simulink library "wt_blockset_v3"  (Simulink 6.0)
settings: Solver=ode45  SolverMode=SingleTasking  StartTime=0.0  StopTime=10.0  RelTol=1e-3
undefined symbols (not defined in the file): f1, get, j, Kmode, Type, u0
libraries: simulink_extras x12, simulink3 x5, simulink x4, dspinverses x1, dspmtrx3 x1, dspsnks4 x1
(part 5 of 7)

== system wt_blockset_v3/Mechanical Components/Wind Model ZA-1/Kaimal_Filter_2 ==
  in_1 : Inport  Port=1  LatchInput=off
  Gain : Gain  Gain=trans/sqrt(2)  SaturateOnIntegerOverflow=on
  Transfer Function : TransferFcn  Numerator=[0.0182*c^2 1.3653*c 0.9846]  Denominator=[1.3463*c^2 3.7593*c 1]
  Unit Delay : UnitDelay  SampleTime=T_sample
  out_1 : Outport
  wires:
  Unit Delay/1 -> Transfer Function/1
  Gain/1 -> out_1/1
  in_1/1 -> Unit Delay/1
  Transfer Function/1 -> Gain/1

== system wt_blockset_v3/Mechanical Components/Wind Model ZA-1/Kaimal_Filter_3 ==
  in_1 : Inport  Port=1  LatchInput=off
  Gain : Gain  Gain=trans/sqrt(2)  SaturateOnIntegerOverflow=on
  Transfer Fcn : TransferFcn  Numerator=[0.0182*c^2 1.3653*c 0.9846]  Denominator=[1.3463*c^2 3.7593*c 1]
  Unit Delay : UnitDelay  SampleTime=T_sample
  out_1 : Outport
  wires:
  Unit Delay/1 -> Transfer Fcn/1
  Gain/1 -> out_1/1
  in_1/1 -> Unit Delay/1
  Transfer Fcn/1 -> Gain/1

== system wt_blockset_v3/Mechanical Components/Wind Model ZA-2/3rd_Harmonic_Filter1 ==
  avg_wind : Inport  Port=1  LatchInput=off
  in_1 : Inport  Port=2  LatchInput=off
  3rd harmonic Filter : Subsystem
  Unit Delay : UnitDelay  SampleTime=T_sample
  out_1 : Outport
  wires:
  Unit Delay/1 -> 3rd harmonic Filter/2(In)
  in_1/1 -> Unit Delay/1
  avg_wind/1 -> 3rd harmonic Filter/1(avg_wind)
  3rd harmonic Filter/1(Out) -> out_1/1

== system wt_blockset_v3/Mechanical Components/Wind Model ZA-2/3rd_Harmonic_Filter2 ==
  avg_wind : Inport  Port=1  LatchInput=off
  in_1 : Inport  Port=2  LatchInput=off
  3rd harmonic Filter : Subsystem
  Unit Delay : UnitDelay  SampleTime=T_sample
  out_1 : Outport
  wires:
  3rd harmonic Filter/1(Out) -> out_1/1
  avg_wind/1 -> 3rd harmonic Filter/1(avg_wind)
  in_1/1 -> Unit Delay/1
  Unit Delay/1 -> 3rd harmonic Filter/2(In)

== system wt_blockset_v3/Mechanical Components/Wind Model ZA-2/Band Limited White Noise ==
  Gain : Gain  Gain=sqrt(noise/T_sample)  SaturateOnIntegerOverflow=on
  S-Function : S-Function  FunctionName=rngen  Parameters=seed
  Zero-Order Hold : ZeroOrderHold  SampleTime=T_sample
  wn : Outport
  wires:
  S-Function/1 -> Zero-Order Hold/1
  Zero-Order Hold/1 -> Gain/1
  Gain/1 -> wn/1

== system wt_blockset_v3/Mechanical Components/Wind Model ZA-2/Band Limited White Noise1 ==
  Gain : Gain  Gain=sqrt(noise/T_sample)  SaturateOnIntegerOverflow=on
  S-Function : S-Function  FunctionName=rngen  Parameters=seed
  Zero-Order Hold : ZeroOrderHold  SampleTime=T_sample
  wn : Outport
  wires:
  Gain/1 -> wn/1
  Zero-Order Hold/1 -> Gain/1
  S-Function/1 -> Zero-Order Hold/1

== system wt_blockset_v3/Mechanical Components/Wind Model ZA-2/Band Limited White Noise2 ==
  Gain : Gain  Gain=sqrt(noise/T_sample)  SaturateOnIntegerOverflow=on
  S-Function : S-Function  FunctionName=rngen  Parameters=seed
  Zero-Order Hold : ZeroOrderHold  SampleTime=T_sample
  wn : Outport
  wires:
  S-Function/1 -> Zero-Order Hold/1
  Zero-Order Hold/1 -> Gain/1
  Gain/1 -> wn/1

== system wt_blockset_v3/Mechanical Components/Wind Model ZA-2/Kaimal_Filter_1 ==
  in_1 : Inport  Port=1  LatchInput=off
  avg_wind : Inport  Port=2  LatchInput=off
  Fcn : Fcn  Expr=turb_int*sqrt(L*u(1))/100/sqrt(2)
  Kaimal Filter : Subsystem
  Product : Product  SaturateOnIntegerOverflow=on
  Unit Delay : UnitDelay  SampleTime=T_sample
  out_1 : Outport
  wires:
  Unit Delay/1 -> Kaimal Filter/2(In)
  in_1/1 -> Unit Delay/1
  avg_wind/1 -> Kaimal Filter/1(avg_wind), Fcn/1
  Fcn/1 -> Product/1
  Kaimal Filter/1(Out) -> Product/2
  Product/1 -> out_1/1

== system wt_blockset_v3/Mechanical Components/Wind Model ZA-2/Kaimal_Filter_2 ==
  avg_wind : Inport  Port=1  LatchInput=off
  in_1 : Inport  Port=2  LatchInput=off
  Fcn : Fcn  Expr=turb_int*sqrt(L*u(1))/100/sqrt(2)
  Kaimal Filter : Subsystem
  Product : Product  SaturateOnIntegerOverflow=on
  Unit Delay : UnitDelay  SampleTime=T_sample
  out_1 : Outport
  wires:
  Product/1 -> out_1/1
  Kaimal Filter/1(Out) -> Product/2
  Fcn/1 -> Product/1
  avg_wind/1 -> Fcn/1, Kaimal Filter/1(avg_wind)
  in_1/1 -> Unit Delay/1
  Unit Delay/1 -> Kaimal Filter/2(In)

== system wt_blockset_v3/Mechanical Components/Wind Model ZA-2/Kaimal_Filter_3 ==
  avg_wind : Inport  Port=1  LatchInput=off
  in_1 : Inport  Port=2  LatchInput=off
  Fcn : Fcn  Expr=turb_int*sqrt(L*u(1))/100/sqrt(2)
  Kaimal Filter : Subsystem
  Product : Product  SaturateOnIntegerOverflow=on
  Unit Delay : UnitDelay  SampleTime=T_sample
  out_1 : Outport
  wires:
  Unit Delay/1 -> Kaimal Filter/2(In)
  in_1/1 -> Unit Delay/1
  avg_wind/1 -> Kaimal Filter/1(avg_wind), Fcn/1
  Fcn/1 -> Product/1
  Kaimal Filter/1(Out) -> Product/2
  Product/1 -> out_1/1

== system wt_blockset_v3/Mechanical Components/Wind Model ZA-2/ZERO_Harmonic_Filter ==
  in_1 : Inport  Port=1  LatchInput=off
  avg_wind : Inport  Port=2  LatchInput=off
  Unit Delay : UnitDelay  SampleTime=T_sample
  ZERO harmonic Filter : Subsystem
  out_1 : Outport
  wires:
  ZERO harmonic Filter/1(Out) -> out_1/1
  avg_wind/1 -> ZERO harmonic Filter/1(avg_wind)
  in_1/1 -> Unit Delay/1
  Unit Delay/1 -> ZERO harmonic Filter/2(In)

== system wt_blockset_v3/Power Converters/3-phase Diode Bridge Rectifier/Diode  State Calculator ==
  note: K = [d1 - d4
      |        d3 - d6
      |         d5 - d2]
  RST : Inport  Port=1  LatchInput=off
  Branch A+ : Subsystem
  Branch A- : Subsystem
  Branch B+ : Subsystem
  Branch B- : Subsystem
  Branch C+ : Subsystem
  Branch C- : Subsystem
  Mux : Mux  Inputs=3
  Sum : Sum  Inputs=+-  SaturateOnIntegerOverflow=on  InputSameDT=on
  Sum1 : Sum  Inputs=+-  SaturateOnIntegerOverflow=on  InputSameDT=on
  Sum2 : Sum  Inputs=+-  SaturateOnIntegerOverflow=on  InputSameDT=on
  K : Outport  InitialOutput=0
  wires:
  RST/1 -> Branch A+/1(RST), Branch B+/1(RST), Branch B-/1(RST), Branch C+/1(RST), Branch C-/1(RST), Branch A-/1(RST)
  Branch A+/1(A) -> Sum/1
  Branch A-/1(A) -> Sum/2
  Branch B+/1(B) -> Sum1/1
  Branch B-/1(B) -> Sum1/2
  Branch C+/1(C) -> Sum2/1
  Branch C-/1(C) -> Sum2/2
  Sum/1 -> Mux/1
  Sum1/1 -> Mux/2
  Sum2/1 -> Mux/3
  Mux/1 -> K/1

== system wt_blockset_v3/Power Converters/Average SVM Strategy/1st quadrant ==
  note: 1st quadrant
  vd : Inport  Port=1  LatchInput=off
  vq : Inport  Port=2  LatchInput=off
  Action Port : ActionPort  InitializeStates=reset
  Gain : Gain  Gain=sqrt(3)  SaturateOnIntegerOverflow=on
  If : If  NumInputs=2  IfExpression=u2 < u1
  Sector 0 : Subsystem  TreatAsAtomicUnit=on
  Sector 1 : Subsystem  TreatAsAtomicUnit=on
  Sum : Sum  Inputs=+|+  SaturateOnIntegerOverflow=on
  duty_ABC : Outport  OutputWhenDisabled=reset  InitialOutput=[0 0 0]
  wires:
  vd/1 -> Gain/1, [vd]
  vq/1 -> If/2, [vq]
  Gain/1 -> If/1
  If/1 -> Sector 0/Action
  [vd] -> Sector 0/1(vd)
  [vq] -> Sector 0/2(vq)
  If/2 -> Sector 1/Action
  [vd] -> Sector 1/1(vd)
  [vq] -> Sector 1/2(vq)
  Sector 1/1(duty_ABC) -> Sum/2
  Sector 0/1(duty_ABC) -> Sum/1
  Sum/1 -> duty_ABC/1

== system wt_blockset_v3/Power Converters/Average SVM Strategy/2nd quadrant ==
  note: 2nd quadrant
  vd : Inport  Port=1  LatchInput=off
  vq : Inport  Port=2  LatchInput=off
  Action Port : ActionPort  InitializeStates=reset
  Abs : Abs  SaturateOnIntegerOverflow=on
  Gain : Gain  Gain=sqrt(3)  SaturateOnIntegerOverflow=on
  If : If  NumInputs=2  IfExpression=u2 < u1
  Sector 1 : Subsystem  TreatAsAtomicUnit=on
  Sector 2 : Subsystem  TreatAsAtomicUnit=on
  Sum : Sum  Inputs=+|+  SaturateOnIntegerOverflow=on
  duty_ABC : Outport  OutputWhenDisabled=reset  InitialOutput=[0 0 0]
  wires:
  Sum/1 -> duty_ABC/1
  Sector 2/1(duty_ABC) -> Sum/1
  Sector 1/1(duty_ABC) -> Sum/2
  [vq] -> Sector 1/2(vq)
  [vd] -> Sector 1/1(vd)
  If/2 -> Sector 1/Action
  [vq] -> Sector 2/2(vq)
  [vd] -> Sector 2/1(vd)
  If/1 -> Sector 2/Action
  vq/1 -> [vq], If/2
  vd/1 -> [vd], Abs/1
  Gain/1 -> If/1
  Abs/1 -> Gain/1

== system wt_blockset_v3/Power Converters/Average SVM Strategy/3rd quadrant ==
  note: 3rd quadrant
  vd : Inport  Port=1  LatchInput=off
  vq : Inport  Port=2  LatchInput=off
  Action Port : ActionPort  InitializeStates=reset
  Abs : Abs  SaturateOnIntegerOverflow=on
  Abs1 : Abs  SaturateOnIntegerOverflow=on
  Gain : Gain  Gain=sqrt(3)  SaturateOnIntegerOverflow=on
  If : If  NumInputs=2  IfExpression=u2 <= u1
  Sector 3 : Subsystem  TreatAsAtomicUnit=on
  Sector 4 : Subsystem  TreatAsAtomicUnit=on
  Sum : Sum  Inputs=+|+  SaturateOnIntegerOverflow=on
  duty_ABC : Outport  OutputWhenDisabled=reset  InitialOutput=[0 0 0]
  wires:
  Sum/1 -> duty_ABC/1
  Sector 3/1(duty_ABC) -> Sum/1
  Sector 4/1(duty_ABC) -> Sum/2
  [vq] -> Sector 4/2(vq)
  [vd] -> Sector 4/1(vd)
  If/2 -> Sector 4/Action
  [vq] -> Sector 3/2(vq)
  [vd] -> Sector 3/1(vd)
  If/1 -> Sector 3/Action
  vq/1 -> [vq], Abs1/1
  vd/1 -> [vd], Abs/1
  Gain/1 -> If/1
  Abs/1 -> Gain/1
  Abs1/1 -> If/2

== system wt_blockset_v3/Power Converters/Average SVM Strategy/4th quadrant ==
  note: 4th quadrant
  vd : Inport  Port=1  LatchInput=off
  vq : Inport  Port=2  LatchInput=off
  Action Port : ActionPort  InitializeStates=reset
  Abs1 : Abs  SaturateOnIntegerOverflow=on
  Gain : Gain  Gain=sqrt(3)  SaturateOnIntegerOverflow=on
  If : If  NumInputs=2  IfExpression=u2 <= u1
  Sector 4 : Subsystem  TreatAsAtomicUnit=on
  Sector 5 : Subsystem  TreatAsAtomicUnit=on
  Sum : Sum  Inputs=+|+  SaturateOnIntegerOverflow=on
  duty_ABC : Outport  OutputWhenDisabled=reset  InitialOutput=[0 0 0]
  wires:
  Abs1/1 -> If/2
  vd/1 -> [vd], Gain/1
  vq/1 -> Abs1/1, [vq]
  If/1 -> Sector 5/Action
  [vd] -> Sector 5/1(vd)
  [vq] -> Sector 5/2(vq)
  If/2 -> Sector 4/Action
  [vd] -> Sector 4/1(vd)
  [vq] -> Sector 4/2(vq)
  Sector 4/1(duty_ABC) -> Sum/2
  Sector 5/1(duty_ABC) -> Sum/1
  Sum/1 -> duty_ABC/1
  Gain/1 -> If/1

== system wt_blockset_v3/Power Converters/Average SVM Strategy/Avoid saturation  ==
  Mux : Mux  Inputs=7
  Sign_vdref : Signum
  Sign_vqref : Signum
  vd : Fcn  Expr=(abs(u[1])>u[6])*((3*u(2)*u[6])/(2*u[5]))+(abs(u[1])<=u[6])*(3*u[1]/2/u[5])
  vq : Fcn  Expr=(abs(u[3])>u[7])*((3*u(4)*u[7])/(2*u[5]))+(abs(u[3])<=u[7])*(3*u[3]/2/u[5])
  tag scope: vd=global, vq=global
  wires:
  [vdref] -> Mux/1, Sign_vdref/1
  Mux/1 -> vd/1, vq/1
  vd/1 -> [vd]
  vq/1 -> [vq]
  Sign_vdref/1 -> Mux/2
  [vqref] -> Mux/3, Sign_vqref/1
  Sign_vqref/1 -> Mux/4
  [vdc] -> Mux/5
  [dlim] -> Mux/6
  [qlim] -> Mux/7

== system wt_blockset_v3/Power Converters/Average SVM Strategy/Weight ==
  Abs : Abs  SaturateOnIntegerOverflow=on
  "Abs " : Abs  SaturateOnIntegerOverflow=on
  Mux : Mux  Inputs=3
  Product : Product  SaturateOnIntegerOverflow=on
  Product1 : Product  SaturateOnIntegerOverflow=on
  weight : Fcn  Expr=u(2)/(sqrt(3)*sqrt(u(1)^2+u(3)^2))
  tag scope: dlim=global, qlim=global
  wires:
  [vdref] -> Mux/1, Product/1
  Mux/1 -> weight/1
  [vdc] -> Mux/2
  [vqref] -> Mux/3, Product1/2
  weight/1 -> Product/2, Product1/1
  Product/1 -> Abs/1
  Product1/1 -> "Abs "/1
  Abs/1 -> [dlim]
  "Abs "/1 -> [qlim]

== system wt_blockset_v3/Power Converters/Average SVM Strategy/capcom duty cycle ==
  duty_ABC : Inport  Port=1  LatchInput=off
  Constant : Constant  Value=0.5
  Sum : Sum  Inputs=|+-  SaturateOnIntegerOverflow=on
  pwm_abc : Outport
  wires:
  Constant/1 -> Sum/2
  Sum/1 -> pwm_abc/1
  duty_ABC/1 -> Sum/1

== system wt_blockset_v3/Power Converters/Average SVM Strategy C_Sfun/capcom duty cycle ==
  duty_ABC : Inport  Port=1  LatchInput=off
  Constant : Constant  Value=0.5
  Sum : Sum  Inputs=|+-  SaturateOnIntegerOverflow=on
  pwm_abc : Outport
  wires:
  Constant/1 -> Sum/2
  Sum/1 -> pwm_abc/1
  duty_ABC/1 -> Sum/1

== system wt_blockset_v3/Power Converters/RMS - Soft Starter/Look-up table extinction angle ==
  firing angle : Inport  Port=1  LatchInput=off
  phase : Inport  Port=2  LatchInput=off
  Extinction angle1 : simulink3/Functions & Tables/Interpolation (n-D) using PreLook-Up  numDimsPopupSelect=2  explicitNumDims=2  table=ext_angle  interpMethod=Linear  extrapMethod=None - Clip  rangeErrorMode=Warning
  Fcn : Fcn  Expr=u(2)*(u(2)>=u(1))+u(1)*(u(2)<u(1))
  Mux : Mux  Inputs=2
  PreLook-Up Index Search2 : simulink3/Functions & Tables/PreLook-Up Index Search  bpData=[0:15:180]  searchMode=Evenly Spaced Points  cacheBpFlag=off  outputFlag=off  extrapMode=Clip to Range  rangeErrorMode=Warning
  PreLook-Up Index Search3 : simulink3/Functions & Tables/PreLook-Up Index Search  bpData=[0:15:90]  searchMode=Evenly Spaced Points  cacheBpFlag=off  outputFlag=off  extrapMode=Clip to Range  rangeErrorMode=Warning
  extinction : Outport
  wires:
  PreLook-Up Index Search3/1 -> Extinction angle1/1
  PreLook-Up Index Search2/1 -> Extinction angle1/2
  phase/1 -> PreLook-Up Index Search3/1, Mux/1
  firing angle/1 -> Mux/2
  Mux/1 -> Fcn/1
  Fcn/1 -> PreLook-Up Index Search2/1
  Extinction angle1/1 -> extinction/1

== system wt_blockset_v3/Power Converters/Sinus PWM/Vtri ==
  Constant1 : Constant
  Constant2 : Constant
  Constant3 : Constant  Value=0
  Fcn : Fcn  Expr=-u(1)*2+1
  Gain : Gain  Gain=fsw2  SaturateOnIntegerOverflow=on
  Gain1 : Gain  Gain=2*fsw2  SaturateOnIntegerOverflow=on
  IC : InitialCondition  Value=1.5
  Integrator : Integrator  ExternalReset=rising  InitialConditionSource=external  InitialCondition=1.5
  Integrator1 : Integrator  ExternalReset=rising
  Pulse Generator : simulink3/Sources/Pulse Generator  period=2/fsw2  duty=50  amplitude=1  start=0.5/fsw2
  Pulse Generator1 : simulink3/Sources/Pulse Generator  period=2/fsw2  duty=50  amplitude=1  start=0
  Relational Operator : RelationalOperator  InputSameDT=on
  Vtri : Outport  InitialOutput=0
  wires:
  Integrator1/1 -> Vtri/1
  Pulse Generator/1 -> Integrator/2
  Constant2/1 -> Gain/1
  Fcn/1 -> Gain1/1
  Relational Operator/1 -> Fcn/1
  Integrator/1 -> Relational Operator/1
  IC/1 -> Integrator/3
  Constant3/1 -> IC/1
  Pulse Generator1/1 -> Integrator1/2
  Gain1/1 -> Integrator1/1
  Gain/1 -> Integrator/1
  Constant1/1 -> Relational Operator/2

== system wt_blockset_v3/Power Converters/Sinus PWM/logical ==
  In1 : Inport  Port=1  LatchInput=off
  Constant : Constant  Value=0
  Hit  Crossing : HitCross  ShowOutputPort=off
  IC : InitialCondition  Value=0
  Relational Operator : RelationalOperator  InputSameDT=on
  Out1 : Outport  InitialOutput=0
  wires:
  IC/1 -> Out1/1
  Constant/1 -> Relational Operator/2
  In1/1 -> Relational Operator/1
  Relational Operator/1 -> IC/1, Hit  Crossing/1

== system wt_blockset_v3/Power Converters/Soft-Starter/S-R flip flop ==
  S : Inport  Port=1  LatchInput=off
  R : Inport  Port=2  LatchInput=off
  Demux : Demux  Outputs=6
  Demux1 : Demux  Outputs=6
  Mux : Mux  Inputs=6
  S-R Flip-Flop1 : Subsystem  mask(SRFlipFlop){initial_condition=init_a}
      mask prompts: initial_condition "Initial condition (state of Q):"
      mask help: S-R Flip-Flop Block
      mask Help:
      | The S-R flip-flop also known as a set-reset flip-flop. This implementation
      | is modeled after an S-R flip-flop constructed using NOR gates. The
      | truth table for this block is:
      | <pre>
      |  S  R   Q  !Q
      |  ----------------
      |  1  0   1  0
      |  0  0   1  0  (after S == 1, R == 0)
      |  0  1   0  1
      |  0  0   0  1  (after S == 0, R == 1)
      |  1  1   0  0
      | </pre>
      | 
      | In an S-R flip-flop that is implemented with NOR gates, when a 1 is
      | applied to both the set and reset inputs, both outputs go to 0. Technically,
      | this state is undefined and is usually avoided. Note, if the flip-flop is
      | implemented with NAND gates, when a 0 is applied to both inputs, both outputs
      | go to 0 and when a 1 is applied to both inputs, the output depends on
      | the previous state of the flip-flop (previous value of Q).
  S-R Flip-Flop2 : Subsystem  mask(SRFlipFlop){initial_condition=init_b}
      mask prompts: initial_condition "Initial condition (state of Q):"
      mask help: S-R Flip-Flop Block
      mask Help:
      | The S-R flip-flop also known as a set-reset flip-flop. This implementation
      | is modeled after an S-R flip-flop constructed using NOR gates. The
      | truth table for this block is:
      | <pre>
      |  S  R   Q  !Q
      |  ----------------
      |  1  0   1  0
      |  0  0   1  0  (after S == 1, R == 0)
      |  0  1   0  1
      |  0  0   0  1  (after S == 0, R == 1)
      |  1  1   0  0
      | </pre>
      | 
      | In an S-R flip-flop that is implemented with NOR gates, when a 1 is
      | applied to both the set and reset inputs, both outputs go to 0. Technically,
      | this state is undefined and is usually avoided. Note, if the flip-flop is
      | implemented with NAND gates, when a 0 is applied to both inputs, both outputs
      | go to 0 and when a 1 is applied to both inputs, the output depends on
      | the previous state of the flip-flop (previous value of Q).
  S-R Flip-Flop3 : Subsystem  mask(SRFlipFlop){initial_condition=init_c}
      mask prompts: initial_condition "Initial condition (state of Q):"
      mask help: S-R Flip-Flop Block
      mask Help:
      | The S-R flip-flop also known as a set-reset flip-flop. This implementation
      | is modeled after an S-R flip-flop constructed using NOR gates. The
      | truth table for this block is:
      | <pre>
      |  S  R   Q  !Q
      |  ----------------
      |  1  0   1  0
      |  0  0   1  0  (after S == 1, R == 0)
      |  0  1   0  1
      |  0  0   0  1  (after S == 0, R == 1)
      |  1  1   0  0
      | </pre>
      | 
      | In an S-R flip-flop that is implemented with NOR gates, when a 1 is
      | applied to both the set and reset inputs, both outputs go to 0. Technically,
      | this state is undefined and is usually avoided. Note, if the flip-flop is
      | implemented with NAND gates, when a 0 is applied to both inputs, both outputs
      | go to 0 and when a 1 is applied to both inputs, the output depends on
      | the previous state of the flip-flop (previous value of Q).
  S-R Flip-Flop4 : Subsystem  mask(SRFlipFlop){initial_condition=init_a}
      mask prompts: initial_condition "Initial condition (state of Q):"
      mask help: S-R Flip-Flop Block
      mask Help:
      | The S-R flip-flop also known as a set-reset flip-flop. This implementation
      | is modeled after an S-R flip-flop constructed using NOR gates. The
      | truth table for this block is:
      | <pre>
      |  S  R   Q  !Q
      |  ----------------
      |  1  0   1  0
      |  0  0   1  0  (after S == 1, R == 0)
      |  0  1   0  1
      |  0  0   0  1  (after S == 0, R == 1)
      |  1  1   0  0
      | </pre>
      | 
      | In an S-R flip-flop that is implemented with NOR gates, when a 1 is
      | applied to both the set and reset inputs, both outputs go to 0. Technically,
      | this state is undefined and is usually avoided. Note, if the flip-flop is
      | implemented with NAND gates, when a 0 is applied to both inputs, both outputs
      | go to 0 and when a 1 is applied to both inputs, the output depends on
      | the previous state of the flip-flop (previous value of Q).
  S-R Flip-Flop5 : Subsystem  mask(SRFlipFlop){initial_condition=~init_b}
      mask prompts: initial_condition "Initial condition (state of Q):"
      mask help: S-R Flip-Flop Block
      mask Help:
      | The S-R flip-flop also known as a set-reset flip-flop. This implementation
      | is modeled after an S-R flip-flop constructed using NOR gates. The
      | truth table for this block is:
      | <pre>
      |  S  R   Q  !Q
      |  ----------------
      |  1  0   1  0
      |  0  0   1  0  (after S == 1, R == 0)
      |  0  1   0  1
      |  0  0   0  1  (after S == 0, R == 1)
      |  1  1   0  0
      | </pre>
      | 
      | In an S-R flip-flop that is implemented with NOR gates, when a 1 is
      | applied to both the set and reset inputs, both outputs go to 0. Technically,
      | this state is undefined and is usually avoided. Note, if the flip-flop is
      | implemented with NAND gates, when a 0 is applied to both inputs, both outputs
      | go to 0 and when a 1 is applied to both inputs, the output depends on
      | the previous state of the flip-flop (previous value of Q).
  S-R Flip-Flop6 : Subsystem  mask(SRFlipFlop){initial_condition=~init_c}
      mask prompts: initial_condition "Initial condition (state of Q):"
      mask help: S-R Flip-Flop Block
      mask Help:
      | The S-R flip-flop also known as a set-reset flip-flop. This implementation
      | is modeled after an S-R flip-flop constructed using NOR gates. The
      | truth table for this block is:
      | <pre>
      |  S  R   Q  !Q
      |  ----------------
      |  1  0   1  0
      |  0  0   1  0  (after S == 1, R == 0)
      |  0  1   0  1
      |  0  0   0  1  (after S == 0, R == 1)
      |  1  1   0  0
      | </pre>
      | 
      | In an S-R flip-flop that is implemented with NOR gates, when a 1 is
      | applied to both the set and reset inputs, both outputs go to 0. Technically,
      | this state is undefined and is usually avoided. Note, if the flip-flop is
      | implemented with NAND gates, when a 0 is applied to both inputs, both outputs
      | go to 0 and when a 1 is applied to both inputs, the output depends on
      | the previous state of the flip-flop (previous value of Q).
  Terminator{,1..5} (6 alike) : Terminator
  Q : Outport
  wires:
  S-R Flip-Flop6/2(!Q) -> Terminator5/1
  S-R Flip-Flop5/2(!Q) -> Terminator4/1
  S-R Flip-Flop4/2(!Q) -> Terminator3/1
  S-R Flip-Flop3/2(!Q) -> Terminator2/1
  S-R Flip-Flop2/2(!Q) -> Terminator1/1
  S-R Flip-Flop1/1(Q) -> Mux/1
  S-R Flip-Flop2/1(Q) -> Mux/2
  S-R Flip-Flop3/1(Q) -> Mux/3
  S-R Flip-Flop4/1(Q) -> Mux/4
  S-R Flip-Flop5/1(Q) -> Mux/5
  Mux/1 -> Q/1
  S-R Flip-Flop6/1(Q) -> Mux/6
  S-R Flip-Flop1/2(!Q) -> Terminator/1
  Demux/1 -> S-R Flip-Flop1/1(S)
  Demux/2 -> S-R Flip-Flop2/1(S)
  Demux/3 -> S-R Flip-Flop3/1(S)
  Demux/4 -> S-R Flip-Flop4/1(S)
  S/1 -> Demux/1
  Demux/6 -> S-R Flip-Flop6/1(S)
  Demux/5 -> S-R Flip-Flop5/1(S)
  R/1 -> Demux1/1
  Demux1/1 -> S-R Flip-Flop1/2(R)
  Demux1/2 -> S-R Flip-Flop2/2(R)
  Demux1/3 -> S-R Flip-Flop3/2(R)
  Demux1/4 -> S-R Flip-Flop4/2(R)
  Demux1/5 -> S-R Flip-Flop5/2(R)
  Demux1/6 -> S-R Flip-Flop6/2(R)

== system wt_blockset_v3/Power Converters/Soft-Starter/S-R flip flop1 ==
  R : Inport  Port=1  LatchInput=off
  S : Inport  Port=2  LatchInput=off
  Demux : Demux  Outputs=6
  Demux1 : Demux  Outputs=6
  Mux : Mux  Inputs=6
  S-R Flip-Flop1 : Subsystem  mask(SRFlipFlop){initial_condition=0}
      mask prompts: initial_condition "Initial condition (state of Q):"
      mask help: S-R Flip-Flop Block
      mask Help:
      | The S-R flip-flop also known as a set-reset flip-flop. This implementation
      | is modeled after an S-R flip-flop constructed using NOR gates. The
      | truth table for this block is:
      | <pre>
      |  S  R   Q  !Q
      |  ----------------
      |  1  0   1  0
      |  0  0   1  0  (after S == 1, R == 0)
      |  0  1   0  1
      |  0  0   0  1  (after S == 0, R == 1)
      |  1  1   0  0
      | </pre>
      | 
      | In an S-R flip-flop that is implemented with NOR gates, when a 1 is
      | applied to both the set and reset inputs, both outputs go to 0. Technically,
      | this state is undefined and is usually avoided. Note, if the flip-flop is
      | implemented with NAND gates, when a 0 is applied to both inputs, both outputs
      | go to 0 and when a 1 is applied to both inputs, the output depends on
      | the previous state of the flip-flop (previous value of Q).
  S-R Flip-Flop2 : Subsystem  mask(SRFlipFlop){initial_condition=0}
      mask prompts: initial_condition "Initial condition (state of Q):"
      mask help: S-R Flip-Flop Block
      mask Help:
      | The S-R flip-flop also known as a set-reset flip-flop. This implementation
      | is modeled after an S-R flip-flop constructed using NOR gates. The
      | truth table for this block is:
      | <pre>
      |  S  R   Q  !Q
      |  ----------------
      |  1  0   1  0
      |  0  0   1  0  (after S == 1, R == 0)
      |  0  1   0  1
      |  0  0   0  1  (after S == 0, R == 1)
      |  1  1   0  0
      | </pre>
      | 
      | In an S-R flip-flop that is implemented with NOR gates, when a 1 is
      | applied to both the set and reset inputs, both outputs go to 0. Technically,
      | this state is undefined and is usually avoided. Note, if the flip-flop is
      | implemented with NAND gates, when a 0 is applied to both inputs, both outputs
      | go to 0 and when a 1 is applied to both inputs, the output depends on
      | the previous state of the flip-flop (previous value of Q).
  S-R Flip-Flop3 : Subsystem  mask(SRFlipFlop){initial_condition=0}
      mask prompts: initial_condition "Initial condition (state of Q):"
      mask help: S-R Flip-Flop Block
      mask Help:
      | The S-R flip-flop also known as a set-reset flip-flop. This implementation
      | is modeled after an S-R flip-flop constructed using NOR gates. The
      | truth table for this block is:
      | <pre>
      |  S  R   Q  !Q
      |  ----------------
      |  1  0   1  0
      |  0  0   1  0  (after S == 1, R == 0)
      |  0  1   0  1
      |  0  0   0  1  (after S == 0, R == 1)
      |  1  1   0  0
      | </pre>
      | 
      | In an S-R flip-flop that is implemented with NOR gates, when a 1 is
      | applied to both the set and reset inputs, both outputs go to 0. Technically,
      | this state is undefined and is usually avoided. Note, if the flip-flop is
      | implemented with NAND gates, when a 0 is applied to both inputs, both outputs
      | go to 0 and when a 1 is applied to both inputs, the output depends on
      | the previous state of the flip-flop (previous value of Q).
  S-R Flip-Flop4 : Subsystem  mask(SRFlipFlop){initial_condition=0}
      mask prompts: initial_condition "Initial condition (state of Q):"
      mask help: S-R Flip-Flop Block
      mask Help:
      | The S-R flip-flop also known as a set-reset flip-flop. This implementation
      | is modeled after an S-R flip-flop constructed using NOR gates. The
      | truth table for this block is:
      | <pre>
      |  S  R   Q  !Q
      |  ----------------
      |  1  0   1  0
      |  0  0   1  0  (after S == 1, R == 0)
      |  0  1   0  1
      |  0  0   0  1  (after S == 0, R == 1)
      |  1  1   0  0
      | </pre>
      | 
      | In an S-R flip-flop that is implemented with NOR gates, when a 1 is
      | applied to both the set and reset inputs, both outputs go to 0. Technically,
      | this state is undefined and is usually avoided. Note, if the flip-flop is
      | implemented with NAND gates, when a 0 is applied to both inputs, both outputs
      | go to 0 and when a 1 is applied to both inputs, the output depends on
      | the previous state of the flip-flop (previous value of Q).
  S-R Flip-Flop5 : Subsystem  mask(SRFlipFlop){initial_condition=0}
      mask prompts: initial_condition "Initial condition (state of Q):"
      mask help: S-R Flip-Flop Block
      mask Help:
      | The S-R flip-flop also known as a set-reset flip-flop. This implementation
      | is modeled after an S-R flip-flop constructed using NOR gates. The
      | truth table for this block is:
      | <pre>
      |  S  R   Q  !Q
      |  ----------------
      |  1  0   1  0
      |  0  0   1  0  (after S == 1, R == 0)
      |  0  1   0  1
      |  0  0   0  1  (after S == 0, R == 1)
      |  1  1   0  0
      | </pre>
      | 
      | In an S-R flip-flop that is implemented with NOR gates, when a 1 is
      | applied to both the set and reset inputs, both outputs go to 0. Technically,
      | this state is undefined and is usually avoided. Note, if the flip-flop is
      | implemented with NAND gates, when a 0 is applied to both inputs, both outputs
      | go to 0 and when a 1 is applied to both inputs, the output depends on
      | the previous state of the flip-flop (previous value of Q).
  S-R Flip-Flop6 : Subsystem  mask(SRFlipFlop){initial_condition=0}
      mask prompts: initial_condition "Initial condition (state of Q):"
      mask help: S-R Flip-Flop Block
      mask Help:
      | The S-R flip-flop also known as a set-reset flip-flop. This implementation
      | is modeled after an S-R flip-flop constructed using NOR gates. The
      | truth table for this block is:
      | <pre>
      |  S  R   Q  !Q
      |  ----------------
      |  1  0   1  0
      |  0  0   1  0  (after S == 1, R == 0)
      |  0  1   0  1
      |  0  0   0  1  (after S == 0, R == 1)
      |  1  1   0  0
      | </pre>
      | 
      | In an S-R flip-flop that is implemented with NOR gates, when a 1 is
      | applied to both the set and reset inputs, both outputs go to 0. Technically,
      | this state is undefined and is usually avoided. Note, if the flip-flop is
      | implemented with NAND gates, when a 0 is applied to both inputs, both outputs
      | go to 0 and when a 1 is applied to both inputs, the output depends on
      | the previous state of the flip-flop (previous value of Q).
  Terminator{,1..5} (6 alike) : Terminator
  Q : Outport
  wires:
  Demux1/6 -> S-R Flip-Flop6/2(R)
  Demux1/5 -> S-R Flip-Flop5/2(R)
  Demux1/4 -> S-R Flip-Flop4/2(R)
  Demux1/3 -> S-R Flip-Flop3/2(R)
  Demux1/2 -> S-R Flip-Flop2/2(R)
  Demux1/1 -> S-R Flip-Flop1/2(R)
  R/1 -> Demux1/1
  Demux/5 -> S-R Flip-Flop5/1(S)
  Demux/6 -> S-R Flip-Flop6/1(S)
  S/1 -> Demux/1
  Demux/4 -> S-R Flip-Flop4/1(S)
  Demux/3 -> S-R Flip-Flop3/1(S)
  Demux/2 -> S-R Flip-Flop2/1(S)
  Demux/1 -> S-R Flip-Flop1/1(S)
  S-R Flip-Flop1/2(!Q) -> Terminator/1
  S-R Flip-Flop6/1(Q) -> Mux/6
  Mux/1 -> Q/1
  S-R Flip-Flop5/1(Q) -> Mux/5
  S-R Flip-Flop4/1(Q) -> Mux/4
  S-R Flip-Flop3/1(Q) -> Mux/3
  S-R Flip-Flop2/1(Q) -> Mux/2
  S-R Flip-Flop1/1(Q) -> Mux/1
  S-R Flip-Flop2/2(!Q) -> Terminator1/1
  S-R Flip-Flop3/2(!Q) -> Terminator2/1
  S-R Flip-Flop4/2(!Q) -> Terminator3/1
  S-R Flip-Flop5/2(!Q) -> Terminator4/1
  S-R Flip-Flop6/2(!Q) -> Terminator5/1

== system wt_blockset_v3/Power Converters/Switching PWM Strategy/capcom ==
  duty_abc : Inport  Port=1  LatchInput=off
  Reshape : simulink/Math Operations/Reshape  OutputDimensionality=1-D array  OutputDimensions=[1,1]
  Sum : Sum  Inputs=-+  SaturateOnIntegerOverflow=on  InputSameDT=on
  Vtri1 : Subsystem  mask{fsw=carrier}
      mask prompts: fsw "switching frequency"
      mask init:
      | fsw2=fsw*2;
      | x=[0 1/4 3/4 1];
      | y=[0 -1     1    0];
      mask Display: plot([x  x+1 ],[y y])
  pulses : Subsystem
      mask init:
      | x=[-5 0 0 5];
      | y=[ 0 0 1 1];
      mask Display: plot(x,y)
  S_ABC : Outport
  wires:
  Reshape/1 -> S_ABC/1  "q"
  Sum/1 -> pulses/1(In1)
  duty_abc/1 -> Sum/2  "Vcontrol"
  Vtri1/1(Vtri) -> Sum/1  "Vtri"
  pulses/1(Out1) -> Reshape/1  "q"

== system wt_blockset_v3/Power Converters/Switching PWM Strategy/dead_time_A ==
  pwm_A : Inport  Port=1  LatchInput=off
  Data Type Conversion : DataTypeConversion  OutDataTypeMode=double  SaturateOnIntegerOverflow=on  RndMeth=Zero
  Data Type Conversion1 : DataTypeConversion  OutDataTypeMode=boolean  SaturateOnIntegerOverflow=on  RndMeth=Zero
  Data Type Conversion2 : DataTypeConversion  OutDataTypeMode=boolean  SaturateOnIntegerOverflow=on  RndMeth=Zero
  Logical Operator : Logic
  Transport Delay : TransportDelay  DelayTime=dead_time  BufferSize=8192
  S_A : Outport
  wires:
  Logical Operator/1 -> Data Type Conversion/1
  pwm_A/1 -> Transport Delay/1, Data Type Conversion1/1
  Transport Delay/1 -> Data Type Conversion2/1
  Data Type Conversion/1 -> S_A/1
  Data Type Conversion1/1 -> Logical Operator/1
  Data Type Conversion2/1 -> Logical Operator/2

== system wt_blockset_v3/Power Converters/Switching PWM Strategy/pulse dropping ==
  duty_ABC : Inport  Port=1  LatchInput=off
  A : Fcn  Expr=(mpw*(u(1)<=mpw)+u(1)*(u(1)>mpw))*(dp==0)+u(1)*(dp==1)
  B : Fcn  Expr=(mpw*(u(2)<=mpw)+u(2)*(u(2)>mpw))*(dp==0)+u(2)*(dp==1)
  C : Fcn  Expr=(mpw*(u(3)<=mpw)+u(3)*(u(3)>mpw))*(dp==0)+u(3)*(dp==1)
  Mux2 : Mux  Inputs=3
  duty_abc : Outport
  wires:
  A/1 -> Mux2/1
  Mux2/1 -> duty_abc/1
  duty_ABC/1 -> A/1, B/1, C/1
  B/1 -> Mux2/2
  C/1 -> Mux2/3

== system wt_blockset_v3/Power Converters/Switching SVM Strategy/1st quadrant ==
  note: 1st quadrant
  vd : Inport  Port=1  LatchInput=off
  vq : Inport  Port=2  LatchInput=off
  Action Port : ActionPort  InitializeStates=reset
  Gain : Gain  Gain=sqrt(3)  SaturateOnIntegerOverflow=on
  If : If  NumInputs=2  IfExpression=u2 < u1
  Sector 0 : Subsystem  TreatAsAtomicUnit=on
  Sector 1 : Subsystem  TreatAsAtomicUnit=on
  Sum : Sum  Inputs=+|+  SaturateOnIntegerOverflow=on
  duty_ABC : Outport  OutputWhenDisabled=reset  InitialOutput=[0 0 0]
  wires:
  vd/1 -> Gain/1, [vd]
  vq/1 -> If/2, [vq]
  Gain/1 -> If/1
  If/1 -> Sector 0/Action
  [vd] -> Sector 0/1(vd)
  [vq] -> Sector 0/2(vq)
  If/2 -> Sector 1/Action
  [vd] -> Sector 1/1(vd)
  [vq] -> Sector 1/2(vq)
  Sector 1/1(duty_ABC) -> Sum/2
  Sector 0/1(duty_ABC) -> Sum/1
  Sum/1 -> duty_ABC/1

== system wt_blockset_v3/Power Converters/Switching SVM Strategy/2nd quadrant ==
  note: 2nd quadrant
  vd : Inport  Port=1  LatchInput=off
  vq : Inport  Port=2  LatchInput=off
  Action Port : ActionPort  InitializeStates=reset
  Abs : Abs  SaturateOnIntegerOverflow=on
  Gain : Gain  Gain=sqrt(3)  SaturateOnIntegerOverflow=on
  If : If  NumInputs=2  IfExpression=u2 < u1
  Sector 1 : Subsystem  TreatAsAtomicUnit=on
  Sector 2 : Subsystem  TreatAsAtomicUnit=on
  Sum : Sum  Inputs=+|+  SaturateOnIntegerOverflow=on
  duty_ABC : Outport  OutputWhenDisabled=reset  InitialOutput=[0 0 0]
  wires:
  Sum/1 -> duty_ABC/1
  Sector 2/1(duty_ABC) -> Sum/1
  Sector 1/1(duty_ABC) -> Sum/2
  [vq] -> Sector 1/2(vq)
  [vd] -> Sector 1/1(vd)
  If/2 -> Sector 1/Action
  [vq] -> Sector 2/2(vq)
  [vd] -> Sector 2/1(vd)
  If/1 -> Sector 2/Action
  vq/1 -> [vq], If/2
  vd/1 -> [vd], Abs/1
  Gain/1 -> If/1
  Abs/1 -> Gain/1

== system wt_blockset_v3/Power Converters/Switching SVM Strategy/3rd quadrant ==
  note: 3rd quadrant
  vd : Inport  Port=1  LatchInput=off
  vq : Inport  Port=2  LatchInput=off
  Action Port : ActionPort  InitializeStates=reset
  Abs : Abs  SaturateOnIntegerOverflow=on
  Abs1 : Abs  SaturateOnIntegerOverflow=on
  Gain : Gain  Gain=sqrt(3)  SaturateOnIntegerOverflow=on
  If : If  NumInputs=2  IfExpression=u2 <= u1
  Sector 3 : Subsystem  TreatAsAtomicUnit=on
  Sector 4 : Subsystem  TreatAsAtomicUnit=on
  Sum : Sum  Inputs=+|+  SaturateOnIntegerOverflow=on
  duty_ABC : Outport  OutputWhenDisabled=reset  InitialOutput=[0 0 0]
  wires:
  Sum/1 -> duty_ABC/1
  Sector 3/1(duty_ABC) -> Sum/1
  Sector 4/1(duty_ABC) -> Sum/2
  [vq] -> Sector 4/2(vq)
  [vd] -> Sector 4/1(vd)
  If/2 -> Sector 4/Action
  [vq] -> Sector 3/2(vq)
  [vd] -> Sector 3/1(vd)
  If/1 -> Sector 3/Action
  vq/1 -> [vq], Abs1/1
  vd/1 -> [vd], Abs/1
  Gain/1 -> If/1
  Abs/1 -> Gain/1
  Abs1/1 -> If/2

== system wt_blockset_v3/Power Converters/Switching SVM Strategy/4th quadrant ==
  note: 4th quadrant
  vd : Inport  Port=1  LatchInput=off
  vq : Inport  Port=2  LatchInput=off
  Action Port : ActionPort  InitializeStates=reset
  Abs1 : Abs  SaturateOnIntegerOverflow=on
  Gain : Gain  Gain=sqrt(3)  SaturateOnIntegerOverflow=on
  If : If  NumInputs=2  IfExpression=u2 <= u1
  Sector 4 : Subsystem  TreatAsAtomicUnit=on
  Sector 5 : Subsystem  TreatAsAtomicUnit=on
  Sum : Sum  Inputs=+|+  SaturateOnIntegerOverflow=on
  duty_ABC : Outport  OutputWhenDisabled=reset  InitialOutput=[0 0 0]
  wires:
  Abs1/1 -> If/2
  vd/1 -> [vd], Gain/1
  vq/1 -> Abs1/1, [vq]
  If/1 -> Sector 5/Action
  [vd] -> Sector 5/1(vd)
  [vq] -> Sector 5/2(vq)
  If/2 -> Sector 4/Action
  [vd] -> Sector 4/1(vd)
  [vq] -> Sector 4/2(vq)
  Sector 4/1(duty_ABC) -> Sum/2
  Sector 5/1(duty_ABC) -> Sum/1
  Sum/1 -> duty_ABC/1
  Gain/1 -> If/1

== system wt_blockset_v3/Power Converters/Switching SVM Strategy/Avoid saturation  ==
  Mux : Mux  Inputs=7
  Sign_vdref : Signum
  Sign_vqref : Signum
  vd : Fcn  Expr=(abs(u[1])>u[6])*((3*u(2)*u[6])/(2*u[5]))+(abs(u[1])<=u[6])*(3*u[1]/2/u[5])
  vq : Fcn  Expr=(abs(u[3])>u[7])*((3*u(4)*u[7])/(2*u[5]))+(abs(u[3])<=u[7])*(3*u[3]/2/u[5])
  tag scope: vd=global, vq=global
  wires:
  [vdref] -> Mux/1, Sign_vdref/1
  Mux/1 -> vd/1, vq/1
  vd/1 -> [vd]
  vq/1 -> [vq]
  Sign_vdref/1 -> Mux/2
  [vqref] -> Mux/3, Sign_vqref/1
  Sign_vqref/1 -> Mux/4
  [vdc] -> Mux/5
  [dlim] -> Mux/6
  [qlim] -> Mux/7

== system wt_blockset_v3/Power Converters/Switching SVM Strategy/Weight ==
  Abs : Abs  SaturateOnIntegerOverflow=on
  "Abs " : Abs  SaturateOnIntegerOverflow=on
  Mux : Mux  Inputs=3
  Product : Product  SaturateOnIntegerOverflow=on
  Product1 : Product  SaturateOnIntegerOverflow=on
  weight : Fcn  Expr=u(2)/(sqrt(3)*sqrt(u(1)^2+u(3)^2))
  tag scope: dlim=global, qlim=global
  wires:
  [vdref] -> Mux/1, Product/1
  Mux/1 -> weight/1
  [vdc] -> Mux/2
  [vqref] -> Mux/3, Product1/2
  weight/1 -> Product/2, Product1/1
  Product/1 -> Abs/1
  Product1/1 -> "Abs "/1
  Abs/1 -> [dlim]
  "Abs "/1 -> [qlim]

== system wt_blockset_v3/Power Converters/Switching SVM Strategy/capcom duty cycle -> 0..1 ==
  duty_ABC : Inport  Port=1  LatchInput=off
  Clock : Clock
  Math Function : Math  Operator=rem  SaturateOnIntegerOverflow=on
  Mux : Mux  Inputs=[3 1]
  Mux2 : Mux  Inputs=3
  Switch_A : Fcn  Expr=(u[4]>=0.5*Tsw*(1-u[1]))*(u[4]<=0.5*Tsw*(1+u[1]))
  Switch_B : Fcn  Expr=(u(4)>=0.5*Tsw*(1-u(2)))*(u(4)<=0.5*Tsw*(1+u(2)))
  Switch_C : Fcn  Expr=(u(4)>=0.5*Tsw*(1-u(3)))*(u(4)<=0.5*Tsw*(1+u(3)))
  Tsw : Constant  Value=Tsw
  pwm_abc : Outport
  wires:
  Mux/1 -> Switch_C/1, Switch_A/1, Switch_B/1
  Math Function/1 -> Mux/2
  Clock/1 -> Math Function/1
  duty_ABC/1 -> Mux/1
  Tsw/1 -> Math Function/2
  Switch_A/1 -> Mux2/1
  Switch_B/1 -> Mux2/2
  Switch_C/1 -> Mux2/3
  Mux2/1 -> pwm_abc/1

== system wt_blockset_v3/Power Converters/Switching SVM Strategy/dead_time_ABC ==
  pwm_ABC : Inport  Port=1  LatchInput=off
  Data Type Conversion : DataTypeConversion  OutDataTypeMode=double  SaturateOnIntegerOverflow=on  RndMeth=Zero
  Data Type Conversion1 : DataTypeConversion  OutDataTypeMode=boolean  SaturateOnIntegerOverflow=on  RndMeth=Zero
  Data Type Conversion2 : DataTypeConversion  OutDataTypeMode=boolean  SaturateOnIntegerOverflow=on  RndMeth=Zero
  Logical Operator : Logic
  Transport Delay : TransportDelay  DelayTime=dead_time  BufferSize=8192
  S_ABC : Outport
  wires:
  Logical Operator/1 -> Data Type Conversion/1
  pwm_ABC/1 -> Transport Delay/1, Data Type Conversion1/1
  Transport Delay/1 -> Data Type Conversion2/1
  Data Type Conversion/1 -> S_ABC/1
  Data Type Conversion1/1 -> Logical Operator/1
  Data Type Conversion2/1 -> Logical Operator/2

== system wt_blockset_v3/Power Converters/Switching SVM Strategy/pulse dropping ==
  duty_ABC : Inport  Port=1  LatchInput=off
  A : Fcn  Expr=(mpw*(u(1)<=mpw)+u(1)*(u(1)>mpw))*(dp==0)+u(1)*(dp==1)
  B : Fcn  Expr=(mpw*(u(2)<=mpw)+u(2)*(u(2)>mpw))*(dp==0)+u(2)*(dp==1)
  C : Fcn  Expr=(mpw*(u(3)<=mpw)+u(3)*(u(3)>mpw))*(dp==0)+u(3)*(dp==1)
  Mux2 : Mux  Inputs=3
  duty_abc : Outport
  wires:
  A/1 -> Mux2/1
  Mux2/1 -> duty_abc/1
  duty_ABC/1 -> A/1, B/1, C/1
  B/1 -> Mux2/2
  C/1 -> Mux2/3

== system wt_blockset_v3/Power Converters/Switching SVM Strategy C_Sfun/capcom duty cycle -> 0..1 ==
  duty_ABC : Inport  Port=1  LatchInput=off
  Clock : Clock
  Math Function : Math  Operator=rem  SaturateOnIntegerOverflow=on
  Mux : Mux  Inputs=[3 1]
  Mux2 : Mux  Inputs=3
  Switch_A : Fcn  Expr=(u[4]>=0.5*Tsw*(1-u[1]))*(u[4]<=0.5*Tsw*(1+u[1]))
  Switch_B : Fcn  Expr=(u(4)>=0.5*Tsw*(1-u(2)))*(u(4)<=0.5*Tsw*(1+u(2)))
  Switch_C : Fcn  Expr=(u(4)>=0.5*Tsw*(1-u(3)))*(u(4)<=0.5*Tsw*(1+u(3)))
  Tsw : Constant  Value=Tsw
  pwm_abc : Outport
  wires:
  Mux/1 -> Switch_C/1, Switch_A/1, Switch_B/1
  Math Function/1 -> Mux/2
  Clock/1 -> Math Function/1
  duty_ABC/1 -> Mux/1
  Tsw/1 -> Math Function/2
  Switch_A/1 -> Mux2/1
  Switch_B/1 -> Mux2/2
  Switch_C/1 -> Mux2/3
  Mux2/1 -> pwm_abc/1

== system wt_blockset_v3/Power Converters/Switching SVM Strategy C_Sfun/dead_time_A ==
  pwm_A : Inport  Port=1  LatchInput=off
  Data Type Conversion : DataTypeConversion  OutDataTypeMode=double  SaturateOnIntegerOverflow=on  RndMeth=Zero
  Data Type Conversion1 : DataTypeConversion  OutDataTypeMode=boolean  SaturateOnIntegerOverflow=on  RndMeth=Zero
  Data Type Conversion2 : DataTypeConversion  OutDataTypeMode=boolean  SaturateOnIntegerOverflow=on  RndMeth=Zero
  Logical Operator : Logic
  Transport Delay : TransportDelay  DelayTime=dead_time  BufferSize=8192
  S_A : Outport
  wires:
  Logical Operator/1 -> Data Type Conversion/1
  pwm_A/1 -> Transport Delay/1, Data Type Conversion1/1
  Transport Delay/1 -> Data Type Conversion2/1
  Data Type Conversion/1 -> S_A/1
  Data Type Conversion1/1 -> Logical Operator/1
  Data Type Conversion2/1 -> Logical Operator/2

== system wt_blockset_v3/Power Converters/Switching SVM Strategy C_Sfun/pulse dropping ==
  duty_ABC : Inport  Port=1  LatchInput=off
  A : Fcn  Expr=(mpw*(u(1)<=mpw)+u(1)*(u(1)>mpw))*(dp==0)+u(1)*(dp==1)
  B : Fcn  Expr=(mpw*(u(2)<=mpw)+u(2)*(u(2)>mpw))*(dp==0)+u(2)*(dp==1)
  C : Fcn  Expr=(mpw*(u(3)<=mpw)+u(3)*(u(3)>mpw))*(dp==0)+u(3)*(dp==1)
  Mux2 : Mux  Inputs=3
  duty_abc : Outport
  wires:
  A/1 -> Mux2/1
  Mux2/1 -> duty_abc/1
  duty_ABC/1 -> A/1, B/1, C/1
  B/1 -> Mux2/2
  C/1 -> Mux2/3

== system wt_blockset_v3/Electrical Machinery/C S-Function based  Models/ABC/abc Squirrel Cage Induction Machine/phase ->line ==
  In : Inport  Port=1  LatchInput=off
  Mux1 : Mux  Inputs=3
  iab : Fcn  Expr=u(1)-u(3)
  ibc : Fcn  Expr=u(2)-u(1)
  ica : Fcn  Expr=u(3)-u(2)
  Out : Outport
  wires:
  iab/1 -> Mux1/1
  ibc/1 -> Mux1/2
  ica/1 -> Mux1/3
  Mux1/1 -> Out/1
  In/1 -> iab/1, ibc/1, ica/1

== system wt_blockset_v3/Electrical Machinery/C S-Function based  Models/ABC/abc Wound Rotor Induction Machine/phase ->line1 ==
  In : Inport  Port=1  LatchInput=off
  Mux1 : Mux  Inputs=3
  iab : Fcn  Expr=u(1)-u(2)
  ibc : Fcn  Expr=u(2)-u(3)
  ica : Fcn  Expr=u(3)-u(1)
  Out : Outport
  wires:
  iab/1 -> Mux1/1
  ibc/1 -> Mux1/2
  ica/1 -> Mux1/3
  Mux1/1 -> Out/1
  In/1 -> iab/1, ibc/1, ica/1

== system wt_blockset_v3/Electrical Machinery/Simulink Blocks  based Models/ABC/abc Squirell-Cage Induction Machine/phase ->line ==
  In : Inport  Port=1  LatchInput=off
  Mux1 : Mux  Inputs=3
  iab : Fcn  Expr=u(1)-u(2)
  ibc : Fcn  Expr=u(2)-u(3)
  ica : Fcn  Expr=u(3)-u(1)
  Out : Outport
  wires:
  iab/1 -> Mux1/1
  ibc/1 -> Mux1/2
  ica/1 -> Mux1/3
  Mux1/1 -> Out/1
  In/1 -> iab/1, ibc/1, ica/1

== system wt_blockset_v3/Electrical Machinery/Simulink Blocks  based Models/Permanent Magnet Synchronous Machine with iron losses/2 to 3  ==
  note: General Transformation from
      | 2-phase to 3-phase
  note: created by: PED9-81A
  theta : Inport  Port=1  LatchInput=off
  u : Inport  Port=2  LatchInput=off
  v : Inport  Port=3  LatchInput=off
  Mux : Mux  Inputs=3
  to A : Fcn  Expr=u[1]*cos(u(3))-u(2)*sin(u(3))
  to B : Fcn  Expr=u[1]*cos(u(3)-2*pi/3)-u(2)*sin(u(3)-2*pi/3)
  to C : Fcn  Expr=u[1]*cos(u(3)+2*pi/3)-u(2)*sin(u(3)+2*pi/3)
  A : Outport
  B : Outport  Port=2
  C : Outport  Port=3
  wires:
  to C/1 -> C/1
  to B/1 -> B/1
  to A/1 -> A/1
  Mux/1 -> to C/1, to B/1, to A/1
  u/1 -> Mux/1
  v/1 -> Mux/2
  theta/1 -> Mux/3

== system wt_blockset_v3/Electrical Machinery/Simulink Blocks  based Models/Permanent Magnet Synchronous Machine with iron losses/3 to 2 ==
  note: created by: PED9-81A
  note: General Transformation from
      | 3-phase to 2-phase
  A : Inport  Port=1  LatchInput=off
  B : Inport  Port=2  LatchInput=off
  C : Inport  Port=3  LatchInput=off
  theta : Inport  Port=4  LatchInput=off
  Mux : Mux
  to d : Fcn  Expr=2/3*(u(1)*cos(u(4))+u(2)*cos(u(4)-2*pi/3)+u(3)*cos(u(4)+2*pi/3))
  to q : Fcn  Expr=-2/3*(u(1)*sin(u(4))+u(2)*sin(u(4)-2*pi/3)+u(3)*sin(u(4)+2*pi/3))
  d : Outport
  q : Outport  Port=2
  wires:
  C/1 -> Mux/3
  B/1 -> Mux/2
  A/1 -> Mux/1
  Mux/1 -> to d/1, to q/1
  to d/1 -> d/1
  to q/1 -> q/1
  theta/1 -> Mux/4

== system wt_blockset_v3/Electrical Machinery/Simulink Blocks  based Models/Permanent Magnet Synchronous Machine with iron losses/Measurement Multiplexor ==
  note: Measurement multiplexor
  note: Created by: PED9-81A
  Mux5 : Mux  Inputs=10
      settings: DisplayOption=signals
  m : Outport
  wires:
  [u_abc] -> Mux5/1  "u_abc"
  [u_dq] -> Mux5/2  "u_dq"
  [i_abc] -> Mux5/3  "i_abc"
  [i_dq] -> Mux5/4  "i_dq"
  [phi_dq] -> Mux5/5  "phi_dq"
  [Te] -> Mux5/6  "Te"
  [wr] -> Mux5/7  "wr"
  [theta] -> Mux5/8  "theta"
  [n] -> Mux5/9  "n"
  [delta] -> Mux5/10  "delta"
  Mux5/1 -> m/1

== system wt_blockset_v3/Electrical Machinery/Simulink Blocks  based Models/Permanent Magnet Synchronous Machine with iron losses/PMSM d-q ==
  note: Permanent Magnet Syncronous Machine d-q Model
      | in Rotor Reference Frame with Iron Losses
  note: created by: PED9-81A
  u_d : Inport  Port=1  LatchInput=off
  u_q : Inport  Port=2  LatchInput=off
  omg : Inport  Port=3  LatchInput=off
  1/s : Integrator
  1/s1 : Integrator
  Const : Constant  Value=0
  Const1 : Constant  Value=s
  Iron losses resistance : Subsystem
  Multiport Switch : MultiPortSwitch  Inputs=2  SaturateOnIntegerOverflow=on  InputSameDT=on
  Mux : Mux  Inputs=6
  Te : Fcn  Expr=1.5*p*u(2)*((Ld-Lq)*u(1)+Ke)
  did/dt : Fcn  Expr=1/Ld*(u(3)-(Rs+u[6])*u(1)+Lq*u(5)*u(2))
  diq/dt : Fcn  Expr=1/Lq*(u(4)-(Rs+u[6])*u(2)-Ld*u(5)*u(1)-u(5)*Ke)
  id : Fcn  Expr=u(1)
  iq : Fcn  Expr=u(2)
  phi-d : Fcn  Expr=Ld*u(1)+Ke
  phi-q : Fcn  Expr=Lq*u(2)
  we : Fcn  Expr=u(5)
  i_d : Outport
  i_q : Outport  Port=2
  T_e : Outport  Port=3
  w_r : Outport  Port=4
  phi_d : Outport  Port=5
  phi_q : Outport  Port=6
  wires:
  did/dt/1 -> 1/s/1
  diq/dt/1 -> 1/s1/1
  Te/1 -> T_e/1  "Te"
  id/1 -> i_d/1  "id"
  iq/1 -> i_q/1  "iq"
  we/1 -> w_r/1  "we"
  Mux/1 -> id/1, Te/1, did/dt/1, diq/dt/1, iq/1, we/1, phi-q/1, phi-d/1
  phi-d/1 -> phi_d/1  "phi_d"
  phi-q/1 -> phi_q/1  "phi_q"
  1/s/1 -> Mux/1  "id"
  1/s1/1 -> Mux/2  "iq"
  u_d/1 -> Mux/3  "ud"
  u_q/1 -> Mux/4  "uq"
  Iron losses resistance/1(Ri) -> Multiport Switch/2  "R_i"
  Multiport Switch/1 -> Mux/6  "Ri"
  Const/1 -> Multiport Switch/3
  Const1/1 -> Multiport Switch/1
  omg/1 -> Mux/5, Iron losses resistance/1(wr)

== system wt_blockset_v3/Electrical Machinery/Simulink Blocks  based Models/Permanent Magnet Synchronous Machine with iron losses/Torque angle ==
  note: Torque angle calculation
  note: Created by: PED9-81A
  i_dq : Inport  Port=1  LatchInput=off
  Demux2 : Demux  Outputs=2
  Trigonometric Function3 : Trigonometry  Operator=atan2
  rad>deg : Gain  Gain=180/pi  SaturateOnIntegerOverflow=on
  T-anlge : Outport
  wires:
  Trigonometric Function3/1 -> rad>deg/1  "T-angle"
  i_dq/1 -> Demux2/1  "i_dq"
  Demux2/2 -> Trigonometric Function3/1  "iq"
  Demux2/1 -> Trigonometric Function3/2  "id"
  rad>deg/1 -> T-anlge/1

== system wt_blockset_v3/Electrical Machinery/Simulink Blocks  based Models/RMS Wound Rotor Induction Machine/Impedance Matrix ==
  omg : Inport  Port=1  LatchInput=off
  Matrix Concatenation1 : simulink/Math Operations/Matrix Concatenation  numInports=2  catMethod=Horizontal
  Matrix Concatenation2 : simulink/Math Operations/Matrix Concatenation  numInports=2  catMethod=Horizontal
  Matrix Concatenation3 : simulink/Math Operations/Matrix Concatenation  numInports=2  catMethod=Vertical
  Product : Product  SaturateOnIntegerOverflow=on  InputSameDT=on
  Product1 : Product  SaturateOnIntegerOverflow=on  InputSameDT=on
  Real-Imag to Complex{,1..3} (4 alike) : RealImagToComplex
  Rs : Constant  Value=Rs
  Xm : Constant  Value=Xm
  Xm1 : Constant  Value=Xm
  Xs : Constant  Value=Xs
  d : Constant  Value=0
  d1 : Constant  Value=0
  rotor reactance : Fcn  Expr=Xsgm_r*(abs(u(1))<=sbd)+(Xsgm_r*((kx-1)*abs(u(1))+(1-kx*sbd))/(1-sbd))*(abs(u(1))>sbd)+Xm
  rotor resistance : Fcn  Expr=Rr*(abs(u(1))<=sbd)+(Rr*((kr-1)*abs(u(1))+(1-kr*sbd))/(1-sbd))*(abs(u(1))>sbd)
  slip : Fcn  Expr=1-u(1)/omg_synch
  Z : Outport
  wires:
  Matrix Concatenation3/1 -> Z/1
  Matrix Concatenation1/1 -> Matrix Concatenation3/1
  Matrix Concatenation2/1 -> Matrix Concatenation3/2
  Real-Imag to Complex2/1 -> Matrix Concatenation2/2
  Real-Imag to Complex3/1 -> Matrix Concatenation2/1
  Xm1/1 -> Product1/1
  Product1/1 -> Real-Imag to Complex3/2
  d1/1 -> Real-Imag to Complex3/1
  Product/1 -> Real-Imag to Complex2/2
  d/1 -> Real-Imag to Complex1/1
  Real-Imag to Complex1/1 -> Matrix Concatenation1/2
  Real-Imag to Complex/1 -> Matrix Concatenation1/1
  Xm/1 -> Real-Imag to Complex1/2
  Xs/1 -> Real-Imag to Complex/2
  Rs/1 -> Real-Imag to Complex/1
  rotor resistance/1 -> Real-Imag to Complex2/1  "Rr"
  omg/1 -> slip/1  "slip"
  slip/1 -> Product1/2, Product/2, rotor reactance/1, rotor resistance/1
  rotor reactance/1 -> Product/1  "Xr"
